simulink model "afa_ut"  (Simulink 8.1)
settings: Solver=FixedStepDiscrete  StartTime=0.0  StopTime=50  FixedStep=5e-3  RelTol=1e-3
libraries: siltestlib x10, afa x1, hcu_lib x1
settings Model: Creator=xsellart  LastModifiedBy=tescamilla
settings DataIOCC: SignalLoggingSaveFormat=Dataset
settings OptimizationCC: ExpressionDepthLimit=128
settings DebuggingCC: FcnCallInpInsideContextMsg=EnableAllAsError
settings GRTTargetCC: CombineOutputUpdateFcns=on  GRTInterface=off

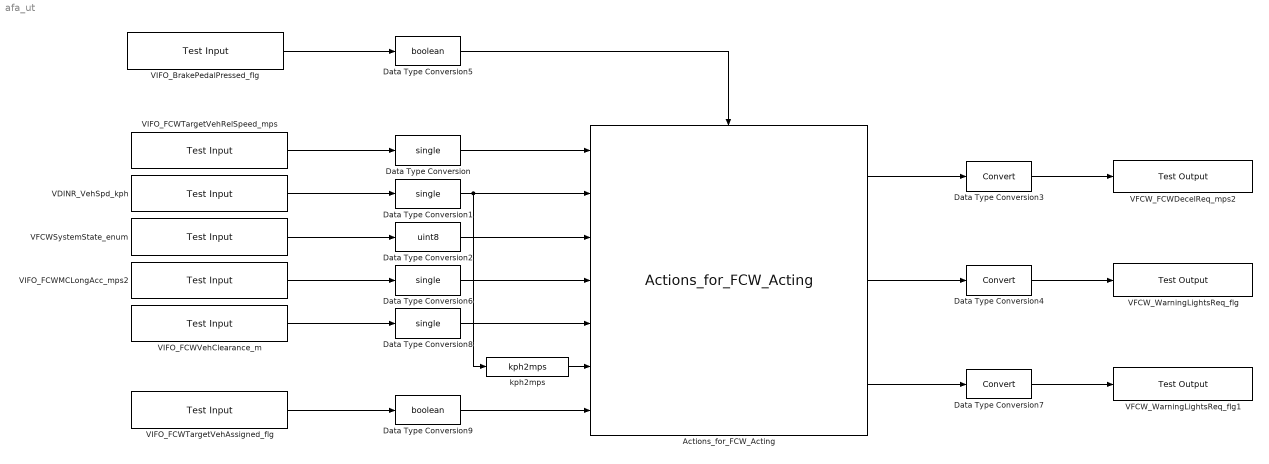
== system afa_ut ==
  Actions_for_FCW_Acting : afa/Actions_for_FCW_Acting
  Data Type Conversion{,1,6,8} (4 alike) : DataTypeConversion  OutDataTypeStr=single
  Data Type Conversion2 : DataTypeConversion  OutDataTypeStr=uint8
  Data Type Conversion3 : DataTypeConversion
  Data Type Conversion4 : DataTypeConversion
  Data Type Conversion5 : DataTypeConversion  OutDataTypeStr=boolean
  Data Type Conversion7 : DataTypeConversion
  Data Type Conversion9 : DataTypeConversion  OutDataTypeStr=boolean
  VDINR_VehSpd_kph : siltestlib/Test Input  varname=VDINR_VehSpd_kph  sampletime=-1
  VFCWSystemState_enum : siltestlib/Test Input  varname=VFCWSystemState_enum  sampletime=-1
  VFCW_FCWDecelReq_mps2 : siltestlib/Test Output  varname=VFCW_FCWDecelReq_mps2  sampletime=-1
  VFCW_WarningLightsReq_flg : siltestlib/Test Output  varname=VFCW_WarningLightsReq_flg  sampletime=-1
  VFCW_WarningLightsReq_flg1 : siltestlib/Test Output  varname=VFCW_FCWHoldReq_flg  sampletime=-1
  VIFO_BrakePedalPressed_flg : siltestlib/Test Input  varname=VFCW_FCWActing_flg  sampletime=-1
  VIFO_FCWMCLongAcc_mps2 : siltestlib/Test Input  varname=VIFO_FCWMCLongAcc_mps2  sampletime=-1
  VIFO_FCWTargetVehAssigned_flg : siltestlib/Test Input  varname=VIFO_FCWTargetVehAssigned_flg  sampletime=-1
  VIFO_FCWTargetVehRelSpeed_mps : siltestlib/Test Input  varname=VIFO_FCWTargetVehRelSpeed_mps  sampletime=-1
  VIFO_FCWVehClearance_m : siltestlib/Test Input  varname=VIFO_FCWVehClearance_m  sampletime=-1
  kph2mps : hcu_lib/kph2mps
  wires:
  VIFO_FCWTargetVehRelSpeed_mps/1 -> Data Type Conversion/1
  VDINR_VehSpd_kph/1 -> Data Type Conversion1/1
  VFCWSystemState_enum/1 -> Data Type Conversion2/1
  Data Type Conversion/1 -> Actions_for_FCW_Acting/1
  Data Type Conversion2/1 -> Actions_for_FCW_Acting/3
  Actions_for_FCW_Acting/1 -> Data Type Conversion3/1
  Data Type Conversion3/1 -> VFCW_FCWDecelReq_mps2/1
  Actions_for_FCW_Acting/2 -> Data Type Conversion4/1
  Data Type Conversion4/1 -> VFCW_WarningLightsReq_flg/1
  Data Type Conversion5/1 -> Actions_for_FCW_Acting/Enable
  VIFO_BrakePedalPressed_flg/1 -> Data Type Conversion5/1
  VIFO_FCWMCLongAcc_mps2/1 -> Data Type Conversion6/1
  Data Type Conversion6/1 -> Actions_for_FCW_Acting/4
  Actions_for_FCW_Acting/3 -> Data Type Conversion7/1
  Data Type Conversion7/1 -> VFCW_WarningLightsReq_flg1/1
  VIFO_FCWVehClearance_m/1 -> Data Type Conversion8/1
  Data Type Conversion8/1 -> Actions_for_FCW_Acting/5
  Data Type Conversion1/1 -> Actions_for_FCW_Acting/2, kph2mps/1
  kph2mps/1 -> Actions_for_FCW_Acting/6
  VIFO_FCWTargetVehAssigned_flg/1 -> Data Type Conversion9/1
  Data Type Conversion9/1 -> Actions_for_FCW_Acting/7
